simulink model "Basic_BMS_model"  (R2017b)
settings: Solver=VariableStepDiscrete  StartTime=0.0  StopTime=10.0  MaxStep=1e-4  RelTol=1e-3
undefined symbols (not defined in the file or in its folder): Ion, Lithium
libraries: powerlib x11, electricdrivelib x3
settings Model: SimulationMode=accelerator  Creator=proso  LastModifiedBy=proso

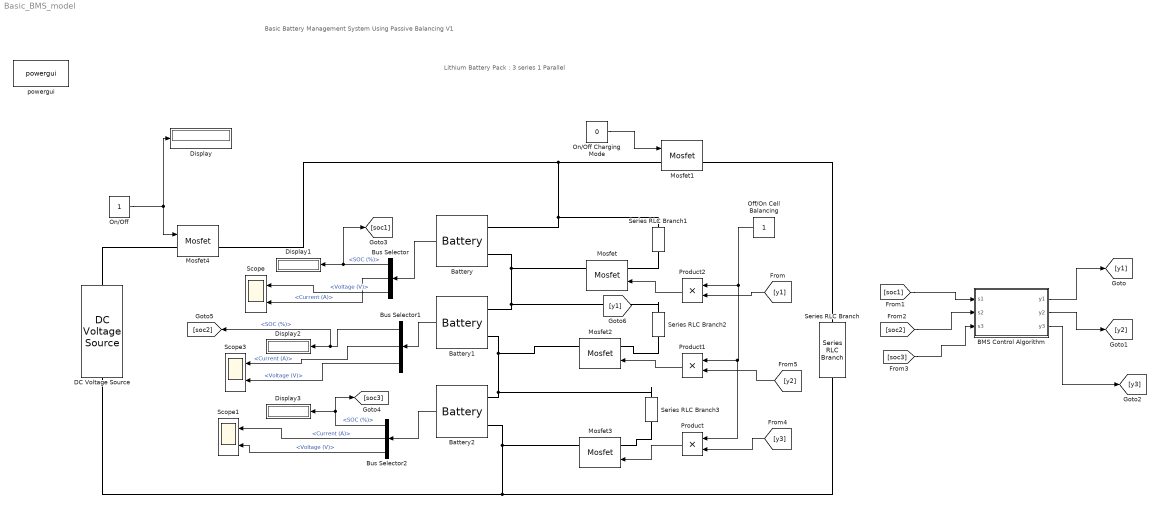
== system Basic_BMS_model ==
  note: Lithium Battery Pack : 3 series 1 Parallel
  note: Basic Battery Management System Using Passive Balancing V1
  BMS Control Algorithm : MATLAB Function  TreatAsAtomicUnit=on
  Battery : electricdrivelib/Extra Sources/Battery  BatType=Lithium-Ion  ShowTempParam=off  ThermalPreset=no  ShowAgeParam=off  NomV=3.7  NomQ=2.6  SOC=54  Batt_Tr=30  PresetModel=off  MaxQ=5.4  MinV=15  FullV=8.3807  Dis_rate=2.3478  R=0.013333  Normal_OP=4.8835  expZone="[7.7788      0.2653]"  current=[6.5 13 32.5]  Units=Time  Tci=20  NomT=20  T2=-30  MaxQ2=4.8  FullV2=7.1  Normal_OP2=5.655  expZone2="[6.58           1]"  Rca=0.6  ti=2000  Dp=0  Neq0=0  Tsim=1e6  Ta1=25  Qeol=5.4*0.9  Reol=0.013333*1.2  Char_age=[2.3478, 3]  Dis_age=[2.3478, 10]  N1=1500  N2=10500  N3=1000  N4=1400  Ta2=45  N5=950
  Battery1 : electricdrivelib/Extra Sources/Battery  BatType=Lithium-Ion  ShowTempParam=off  ThermalPreset=no  ShowAgeParam=off  NomV=3.7  NomQ=2.6  SOC=20  Batt_Tr=30  PresetModel=off  MaxQ=5.4  MinV=15  FullV=8.3807  Dis_rate=2.3478  R=0.013333  Normal_OP=4.8835  expZone="[7.7788      0.2653]"  current=[6.5 13 32.5]  Units=Time  Tci=20  NomT=20  T2=-30  MaxQ2=4.8  FullV2=7.1  Normal_OP2=5.655  expZone2="[6.58           1]"  Rca=0.6  ti=2000  Dp=0  Neq0=0  Tsim=1e6  Ta1=25  Qeol=5.4*0.9  Reol=0.013333*1.2  Char_age=[2.3478, 3]  Dis_age=[2.3478, 10]  N1=1500  N2=10500  N3=1000  N4=1400  Ta2=45  N5=950
  Battery2 : electricdrivelib/Extra Sources/Battery  BatType=Lithium-Ion  ShowTempParam=off  ThermalPreset=no  ShowAgeParam=off  NomV=3.7  NomQ=2.6  SOC=40  Batt_Tr=30  PresetModel=off  MaxQ=5.4  MinV=15  FullV=8.3807  Dis_rate=2.3478  R=0.013333  Normal_OP=4.8835  expZone="[7.7788      0.2653]"  current=[6.5 13 32.5]  Units=Time  Tci=20  NomT=20  T2=-30  MaxQ2=4.8  FullV2=7.1  Normal_OP2=5.655  expZone2="[6.58           1]"  Rca=0.6  ti=2000  Dp=0  Neq0=0  Tsim=1e6  Ta1=25  Qeol=5.4*0.9  Reol=0.013333*1.2  Char_age=[2.3478, 3]  Dis_age=[2.3478, 10]  N1=1500  N2=10500  N3=1000  N4=1400  Ta2=45  N5=950
  Bus Selector : BusSelector  OutputSignals=SOC (%),Current (A),Voltage (V)
  Bus Selector1 : BusSelector  OutputSignals=SOC (%),Current (A),Voltage (V)
  Bus Selector2 : BusSelector  OutputSignals=SOC (%),Current (A),Voltage (V)
  DC Voltage Source : powerlib/Electrical Sources/DC Voltage Source  Amplitude=12  Measurements=None
  Display{,1..3} (4 alike) : Display
  Mosfet{,1..4} (5 alike) : powerlib/Power Electronics/Mosfet  Ron=0.1  Lon=0  Rd=0.01  Vfd=0  IC=0  Rs=1e5  Cs=inf  Measurements=on
  Off/On Cell Balancing : Constant
  On/Off : Constant
  On/Off Charging Mode : Constant  Value=0
  Product : Product
  Product1 : Product
  Product2 : Product
  Scope : Scope  NumInputPorts=2
  Scope1 : Scope  NumInputPorts=2
  Scope3 : Scope  NumInputPorts=2
  Series RLC Branch{,1..3} (4 alike) : powerlib/Elements/Series RLC Branch  LConnTagsString=__new0  RConnTagsString=__new0  BranchType=R  Resistance=1  Inductance=1e-3  SetiL0=off  InitialCurrent=0  Capacitance=1e-6  Setx0=off  InitialVoltage=0  Measurements=None
  powergui : powerlib/powergui  Priority=1  SimulationMode=Discrete  SampleTime=1e-3  frequency=60  Iterations=50  frequencyindice=0  Pbase=100e6  ErrMax=1e-4  UnitsV=kV  UnitsW=MW  buscounter=0  FunctionMessages=off  echomessages=off  EnableUseOfTLC=off  CurrentSourceSwitches=off  DisableSnubberDevices=off  DisableRonSwitches=off  DisableVfSwitches=off  DisplayEquations=off  SolverType=Tustin/Backward Euler (TBE)  Interpol=off  ExternalGateDelay=off  methode=off  Ts=100  x0status=blocks  SPID=on  SwTol=0  HookPort=off  RestoreLinks=warning  ResistiveCurrentMeasurement=off  Frange=[0:2:500]  Ylog=off  Xlog=on  ShowGrid=off  save=off  variable=ZData  structure=0  ZoomFFT=off  StartTime=0.0  cycles=1  DisplayStyle=1  fundamental=60  FreqAxis=off  MaxFrequency=1000  frequencyindicesteady=1  RmsSteady=1  display=off
  wires:
  Off/On Cell Balancing/1 -> Product/1, Product1/1, Product2/1
  Product/1 -> Mosfet3/1
  Product1/1 -> Mosfet2/1
  Product2/1 -> Mosfet/1
  On/Off Charging Mode/1 -> Mosfet1/1
  Battery/1 -> Bus Selector/1
  Battery2/1 -> Bus Selector2/1
  Battery1/1 -> Bus Selector1/1
  BMS Control Algorithm/1(y1) -> [y1]
  On/Off/1 -> Display/1, Mosfet4/1
  Bus Selector/1 -> Display1/1, [soc1]  "<SOC (%)>"
  Bus Selector/2 -> Scope/2  "<Current (A)>"
  Bus Selector/3 -> Scope/1  "<Voltage (V)>"
  [y1] -> Product2/2
  BMS Control Algorithm/2(y2) -> [y2]
  BMS Control Algorithm/3(y3) -> [y3]
  Bus Selector1/1 -> Display2/1, [soc2]  "<SOC (%)>"
  Bus Selector1/2 -> Scope3/1  "<Current (A)>"
  Bus Selector1/3 -> Scope3/2  "<Voltage (V)>"
  Bus Selector2/1 -> Display3/1, [soc3]  "<SOC (%)>"
  Bus Selector2/2 -> Scope1/1  "<Current (A)>"
  Bus Selector2/3 -> Scope1/2  "<Voltage (V)>"
  [soc1] -> BMS Control Algorithm/1(s1)
  [soc2] -> BMS Control Algorithm/2(s2)
  [soc3] -> BMS Control Algorithm/3(s3)
  [y2] -> Product1/2
  [y3] -> Product/2
  connections:
  Mosfet/LConn1 -- Series RLC Branch1/RConn1
  Battery/LConn1 -- Mosfet4/RConn1 -- Mosfet1/LConn1 -- Series RLC Branch1/LConn1
  Mosfet1/RConn1 -- Series RLC Branch/LConn1
  Series RLC Branch/RConn1 -- Mosfet3/RConn1 -- Battery2/LConn2 -- DC Voltage Source/LConn1
  Battery/LConn2 -- Mosfet/RConn1 -- Series RLC Branch2/LConn1 -- Battery1/LConn1
  Mosfet3/LConn1 -- Series RLC Branch3/RConn1
  Battery1/LConn2 -- Mosfet2/RConn1 -- Series RLC Branch3/LConn1 -- Battery2/LConn1
  Mosfet2/LConn1 -- Series RLC Branch2/RConn1
  DC Voltage Source/RConn1 -- Mosfet4/LConn1

== matlab function Basic_BMS_model/BMS Control Algorithm ==
  data: s1 input; y1 output; y2 output; y3 output; s2 input; s3 input
function [y1,y2,y3] = fcn(s1, s2, s3)

s1 = s1*1000;
s2= s2*1000;
s3 = s3*1000;


s1 = int32(s1);
s2 = int32(s2);
s3 = int32(s3);

if s1>s2 || s1>s3
    y1 = 1
else 
    y1 = 0
end

if s2>s1 || s2>s3
    y2 = 1
else 
    y2 = 0
end

if s3>s1 || s3>s2
    y3 = 1
else 
    y3 = 0
end 
    
   
end
